simulink library "stateSpaceMdl"  (R2021b)
settings: Solver=VariableStepAuto  StartTime=0.0  StopTime=10.0  RelTol=1e-3
settings Model: Creator=Lindenmaier László  LastModifiedBy=Lindenmaier László

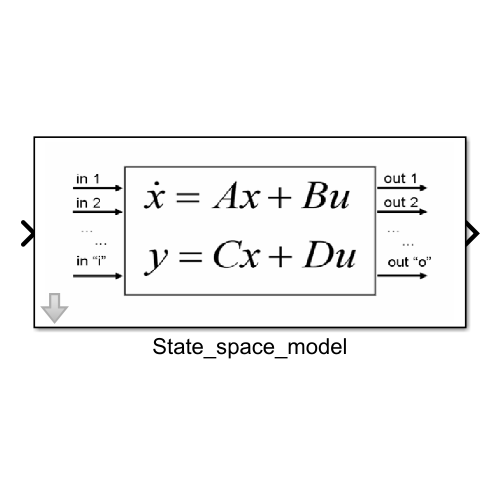
[thumbnail: Simulink's stored preview of the top-level diagram]
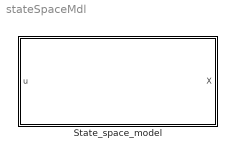
== system stateSpaceMdl ==
  State_space_model : Subsystem  mask{A_in=0, B_in=0}
      mask prompts: A_in "State transition matrix (A)"; B_in "Control matrix (B)"
      mask Display: image('$imagefile'); % Use "Edit Image" on toolstrip to change.

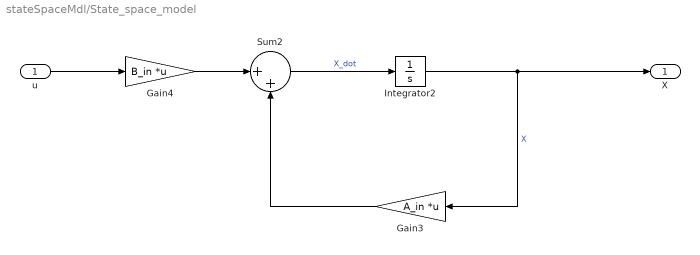
== system stateSpaceMdl/State_space_model ==
  u : Inport
  Gain3 : Gain  Gain=A_in  Multiplication=Matrix(K*u)
  Gain4 : Gain  Gain=B_in  Multiplication=Matrix(K*u)
  Integrator2 : Integrator
  Sum2 : Sum  Inputs=|++
  X : Outport
  wires:
  Gain4/1 -> Sum2/1
  Integrator2/1 -> X/1, Gain3/1  "X"
  Sum2/1 -> Integrator2/1  "X_dot"
  u/1 -> Gain4/1
  Gain3/1 -> Sum2/2
